simulink model "CART3_FAC"  (R2020a)
settings: Solver=ode4  StartTime=0.0  StopTime=TMax  FixedStep=DT  MaxStep=DT  RelTol=1e-3
InitFcn:
  | run('C:\Users\banderso2\Documents\MIRACL\CART3_FAC_paper\CART dependencies\CARTinitFcn.m')
model workspace (MAT data in the model file):
  Vnom = 480
  fnom = 60
undefined symbols (not defined in the file or in its folder): cHinfDiscreteSISO, ctrl, DiscIntNeverNeededParam, DT, GenEff, OutList, strmatch, timer
libraries: cstblocks x7, discretizing x7, powerlib_meascontrol x1
settings Model: Creator=bjonkman  LastModifiedBy=banderso2
settings DataIOCC: LimitDataPoints=on  SaveFormat=Array  SignalLoggingSaveFormat=ModelDataLogs  SaveOutput=off  SaveTime=off  ReturnWorkspaceOutputs=off  SignalLoggingName=sigsOut
settings OptimizationCC: ExpressionDepthLimit=2147483647  LifeSpan=inf
settings DebuggingCC: SaveWithParameterizedLinksMsg=none  MergeDetectMultiDrivingBlocksExec=none  SignalResolutionControl=TryResolveAllWithWarning  MultiTaskDSMMsg=warning  MultiTaskCondExecSysMsg=none  FcnCallInpInsideContextMsg=warning  StateNameClashWarn=warning  SFUnexpectedBacktrackingDiag=warning  SFNoUnconditionalDefaultTransitionDiag=warning  SFExecutionAtInitializationDiag=none  ArithmeticOperatorsInVariantConditions=warning
settings HardwareCC: ProdBitPerPointer=32  ProdBitPerSizeT=32  ProdBitPerPtrDiffT=32  ProdLargestAtomicFloat=None  ProdIntDivRoundTo=Undefined  ProdEndianess=Unspecified  ProdWordSize=32  ProdHWDeviceType=32-bit Generic  TargetUnknown=on
settings ModelReferenceCC: PropagateSignalLabelsOutOfModel=off
settings SFSimCC: SimUseLocalCustomCode=off  CustomCodeUndefinedFunction=UseInterfaceOnly
settings RTWCC: RTWUseLocalCustomCode=off
settings CodeAppCC: StateflowObjectComments=on
settings GRTTargetCC: TargetLangStandard=C89/C90 (ANSI)  CombineOutputUpdateFcns=off  GRTInterface=on
settings ConfigComp: CovMetricSettings=dw  CovHtmlReporting=on  CovSaveCumulativeToWorkspaceVar=on  CovSaveSingleToWorkspaceVar=on  CovExternalEMLEnable=off

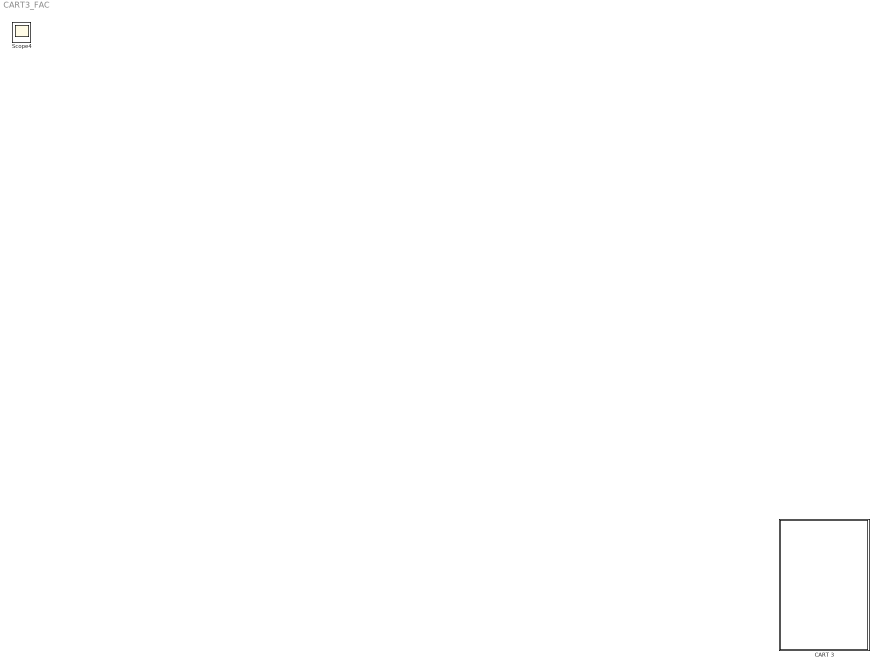
== system CART3_FAC ==
  CART 3 : Subsystem
      mask Display: image('C:\Users\banderso2\Pictures\Saved Pictures\CART3.png'); % Use "Edit Image" on toolstrip to change.
  Scope4 : Scope

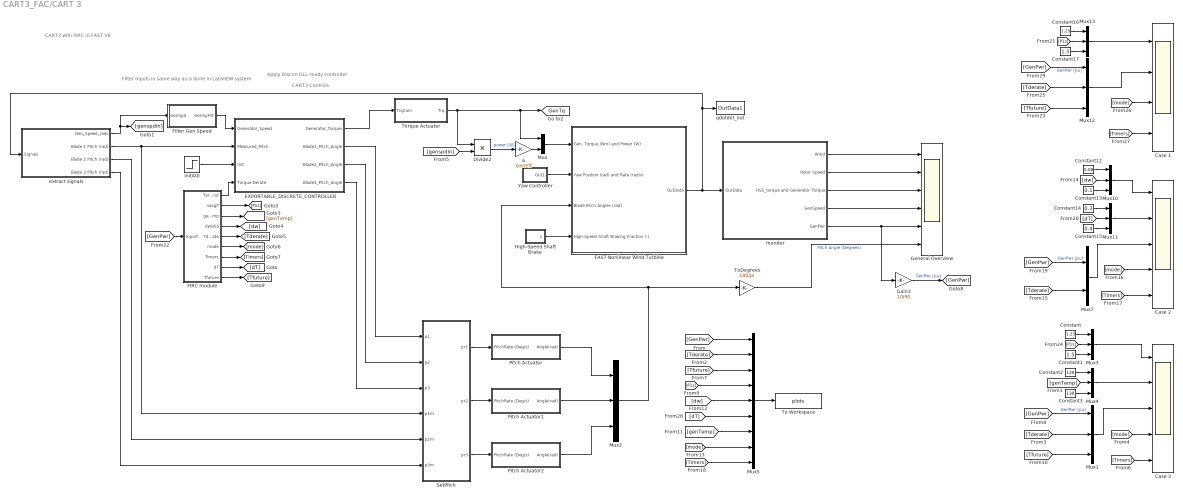
== system CART3_FAC/CART 3 ==
  note: Filter inputs in same way as is done in LabVIEW system
  note: CART3 with FIRC in FAST V8
  note: CART3 Controls
  note: Apply Discon DLL ready controller
  "Case 1 " : Scope  NumInputPorts=4
  Case 2 : Scope  NumInputPorts=5
  Case 3 : Scope  NumInputPorts=5
  Constant : Constant  Value=1.25
  Constant1 : Constant  Value=1.5
  Constant12 : Constant  Value=0.08
  Constant13 : Constant  Value=0.1
  Constant14 : Constant  Value=0.3
  Constant15 : Constant  Value=0.4
  Constant16 : Constant  Value=1.25
  Constant17 : Constant  Value=1.5
  Constant2 : Constant  Value=120
  Constant3 : Constant  Value=130
  Divide2 : Product  Inputs=**
  EXPORTABLE_DISCRETE_CONTROLLER : Subsystem  TreatAsAtomicUnit=on
  FAST Nonlinear Wind Turbine : Subsystem  mask(FAST Nonlinear Wind Turbine){}
      mask help: This block contains the FAST S-Function.
      mask init:
      | clear FAST_SFunc
  "FIRC module " : Subsystem  SystemSampleTime=DT
  Filter Gen Speed : Subsystem  TreatAsAtomicUnit=on
  Gain3 : Gain  Gain=1/590
  General Overview : Scope  NumInputPorts=6
  High-Speed Shaft Brake : Subsystem
  InitAt0 : Step  Time=1/400  SampleTime=DT
  Mux : Mux  Inputs=2
  Mux{1..4,10..13} (8 alike) : Mux  Inputs=3
  Mux5 : Mux  Inputs=9
  Mux7 : Mux  Inputs=2
  Pitch Actuator : Subsystem  TreatAsAtomicUnit=on  SystemSampleTime=DT
  Pitch Actuator1 : Subsystem  TreatAsAtomicUnit=on
  Pitch Actuator2 : Subsystem  TreatAsAtomicUnit=on
  SetPitch : MATLAB Function  TreatAsAtomicUnit=on
  To Workspace : ToWorkspace  VariableName=plots  SaveFormat=Timeseries  SampleTime=-1
  ToDegrees : Gain  Gain=180/pi
  Torque Actuator : Subsystem  TreatAsAtomicUnit=on
  Yaw Controller : Subsystem
  a : Gain  Gain=GenEff
  extract signals : Subsystem
  monitor : Subsystem
  qdotdot_out : ToWorkspace  VariableName=OutData1  SampleTime=-1
  tag scope: GenTq=global
  wires:
  Mux1/1 -> Case 3/3
  "FIRC module "/3(genTemp) -> [genTemp]
  "FIRC module "/5(Tderate) -> [Tderate]
  Divide2/1 -> a/1  "power [W]"
  Yaw Controller/1(Out1) -> FAST Nonlinear Wind Turbine/2(Yaw Position (rad) and Rate (rad/s))
  EXPORTABLE_DISCRETE_CONTROLLER/3(Blade2_Pitch_Angle) -> SetPitch/2(p2)
  Pitch Actuator/1(Angle(rad)) -> Mux2/1
  extract signals/1(Gen_Speed_rads) -> [genspdin], Filter Gen Speed/1(GenSpd)
  ToDegrees/1 -> General Overview/6  "Pitch Angle (Degrees)"
  FAST Nonlinear Wind Turbine/1(OutData) -> monitor/1(OutData), extract signals/1(Signals), qdotdot_out/1
  monitor/4(GenSpeed) -> General Overview/4
  Mux2/1 -> FAST Nonlinear Wind Turbine/3(Blade Pitch Angles (rad)), ToDegrees/1
  SetPitch/2(pr2) -> Pitch Actuator1/1(PitchRate (Deg/s))
  EXPORTABLE_DISCRETE_CONTROLLER/1(Generator_Torque) -> Torque Actuator/1(TrqCom)
  "FIRC module "/4(dwHSS) -> [dw]
  [genspdin] -> Divide2/2
  Pitch Actuator2/1(Angle(rad)) -> Mux2/3
  High-Speed Shaft Brake/1(Out1) -> FAST Nonlinear Wind Turbine/4(High-Speed Shaft Braking Fraction (-))
  SetPitch/3(pr3) -> Pitch Actuator2/1(PitchRate (Deg/s))
  Pitch Actuator1/1(Angle(rad)) -> Mux2/2
  [Timers] -> Case 3/5
  extract signals/2(Blade 1 Pitch (rad)) -> EXPORTABLE_DISCRETE_CONTROLLER/2(Measured_Pitch), SetPitch/4(p1m)
  [mode] -> Case 3/4
  "FIRC module "/6(mode) -> [mode]
  "FIRC module "/2(savgP) -> [P1s]
  EXPORTABLE_DISCRETE_CONTROLLER/2(Blade1_Pitch_Angle) -> SetPitch/1(p1)
  Filter Gen Speed/1(GenSpFilt) -> EXPORTABLE_DISCRETE_CONTROLLER/1(Generator_Speed)
  EXPORTABLE_DISCRETE_CONTROLLER/4(Blade3_Pitch_Angle) -> SetPitch/3(p3)
  Torque Actuator/1(Trq) -> Divide2/1, Mux/1, [GenTq]
  "FIRC module "/1(Torque Command) -> EXPORTABLE_DISCRETE_CONTROLLER/4(Torque Derate)
  "FIRC module "/7(Timers) -> [Timers]
  SetPitch/1(pr1) -> Pitch Actuator/1(PitchRate (Deg/s))
  monitor/3(HSS_torque and Generator Torque) -> General Overview/3
  a/1 -> Mux/2
  monitor/5(GenPwr) -> Gain3/1, General Overview/5
  Mux/1 -> FAST Nonlinear Wind Turbine/1(Gen. Torque (Nm) and Power (W))
  monitor/1(Wind) -> General Overview/1
  InitAt0/1 -> EXPORTABLE_DISCRETE_CONTROLLER/3(Init)
  monitor/2(Rotor Speed) -> General Overview/2
  extract signals/4(Blade 3 Pitch (rad)) -> SetPitch/6(p3m)
  extract signals/3(Blade 2 Pitch (rad)) -> SetPitch/5(p2m)
  "FIRC module "/8(dT) -> [dT]
  Constant/1 -> Mux3/1
  Constant1/1 -> Mux3/3
  Constant2/1 -> Mux4/1
  [genTemp] -> Mux4/2
  Constant3/1 -> Mux4/3
  "FIRC module "/9(Tfuture) -> [Tfuture]
  Mux3/1 -> Case 3/1
  [GenPwr] -> Mux1/1  "GenPwr [pu]"
  [Tderate] -> Mux1/2
  [Tfuture] -> Mux1/3
  Mux11/1 -> Case 2/2
  [Tderate] -> Mux7/2
  [GenPwr] -> Mux7/1  "GenPwr [pu]"
  Constant13/1 -> Mux10/3
  Constant12/1 -> Mux10/1
  Mux7/1 -> Case 2/3
  Constant14/1 -> Mux11/1
  [dw] -> Mux10/2
  [dT] -> Mux11/2
  [Timers] -> Case 2/5
  Constant15/1 -> Mux11/3
  [mode] -> Case 2/4
  Mux10/1 -> Case 2/1
  [Timers] -> "Case 1 "/4
  [Tderate] -> Mux12/2
  [Tfuture] -> Mux12/3
  Mux13/1 -> "Case 1 "/1
  [GenPwr] -> Mux12/1  "GenPwr [pu]"
  Mux12/1 -> "Case 1 "/2
  [mode] -> "Case 1 "/3
  Constant16/1 -> Mux13/1
  [P1s] -> Mux13/2
  Constant17/1 -> Mux13/3
  Mux4/1 -> Case 3/2
  [GenPwr] -> "FIRC module "/1(Inport)
  [P1s] -> Mux3/2
  Gain3/1 -> [GenPwr]  "GenPwr [pu]"
  [GenPwr] -> Mux5/1
  [Tderate] -> Mux5/2
  [Tfuture] -> Mux5/3
  [P1s] -> Mux5/4
  [dw] -> Mux5/5
  [dT] -> Mux5/6
  [genTemp] -> Mux5/7
  [mode] -> Mux5/8
  [Timers] -> Mux5/9
  Mux5/1 -> To Workspace/1

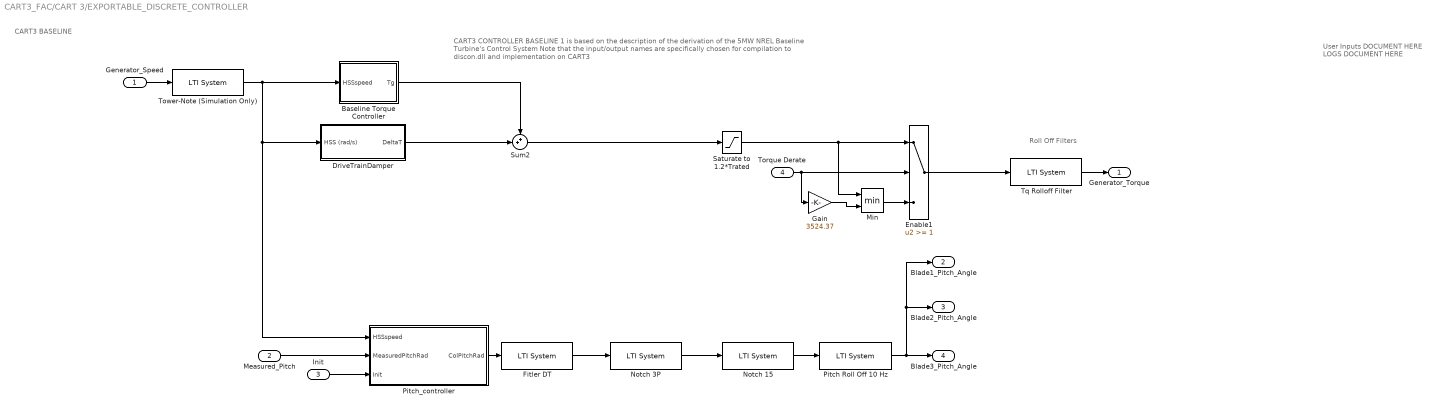
== system CART3_FAC/CART 3/EXPORTABLE_DISCRETE_CONTROLLER ==
  note: CART3 CONTROLLER BASELINE 1 is based on the description of the derivation of the 5MW NREL Baseline Turbine's Control System
      | Note that the input/output names are specifically chosen for compilation to discon.dll and implementation on CART3
  note: Roll Off Filters
  note: User Inputs
      | DOCUMENT HERE
      |
      | LOGS
      | DOCUMENT HERE
  note: CART3 BASELINE
  Generator_Speed : Inport
  Measured_Pitch : Inport  Port=2  PortDimensions=1
  Init : Inport  Port=3  PortDimensions=1
  Torque Derate : Inport  Port=4  PortDimensions=1
  Baseline Torque Controller : Subsystem
  DriveTrainDamper : Subsystem  TreatAsAtomicUnit=on
  Enable1 : Switch  Threshold=1
  Fitler DT : cstblocks/LTI System  sys=FilterDTAdj  IC=[]
  Gain : Gain  Gain=3524.37
  Min : MinMax  Inputs=2
  Notch 15 : cstblocks/LTI System  sys=Notch15  IC=[]
  Notch 3P : cstblocks/LTI System  sys=Notch3PAdj  IC=[]
  Pitch Roll Off 10 Hz : cstblocks/LTI System  sys=PitchRolloff10Hz  IC=[]
  Pitch_controller : Subsystem
  Saturate to 1.2*Trated : Saturate  UpperLimit=1.2*3.5296e+003  LowerLimit=100
  Sum2 : Sum  Inputs=++|
  Tower-Note (Simulation Only) : cstblocks/LTI System  sys=Gen_p9Hz_Notch  IC=[]
  Tq Rolloff Filter : cstblocks/LTI System  sys=TqFilt  IC=[]
  Generator_Torque : Outport
  Blade1_Pitch_Angle : Outport  Port=2  PortDimensions=1
  Blade2_Pitch_Angle : Outport  Port=3  PortDimensions=1
  Blade3_Pitch_Angle : Outport  Port=4  PortDimensions=1
  wires:
  Init/1 -> Pitch_controller/3(Init)
  Generator_Speed/1 -> Tower-Note (Simulation Only)/1
  Fitler DT/1 -> Notch 3P/1
  Notch 3P/1 -> Notch 15/1
  Notch 15/1 -> Pitch Roll Off 10 Hz/1
  Pitch Roll Off 10 Hz/1 -> Blade1_Pitch_Angle/1, Blade2_Pitch_Angle/1, Blade3_Pitch_Angle/1
  Tq Rolloff Filter/1 -> Generator_Torque/1
  Measured_Pitch/1 -> Pitch_controller/2(MeasuredPitchRad)
  Pitch_controller/1(ColPitchRad) -> Fitler DT/1
  Tower-Note (Simulation Only)/1 -> Baseline Torque Controller/1(HSSspeed), Pitch_controller/1(HSSspeed), DriveTrainDamper/1(HSS (rad/s))
  DriveTrainDamper/1(DeltaT) -> Sum2/2
  Baseline Torque Controller/1(Tg) -> Sum2/1
  Sum2/1 -> Saturate to 1.2*Trated/1
  Torque Derate/1 -> Enable1/2, Gain/1
  Saturate to 1.2*Trated/1 -> Min/1, Enable1/1
  Min/1 -> Enable1/3
  Gain/1 -> Min/2
  Enable1/1 -> Tq Rolloff Filter/1

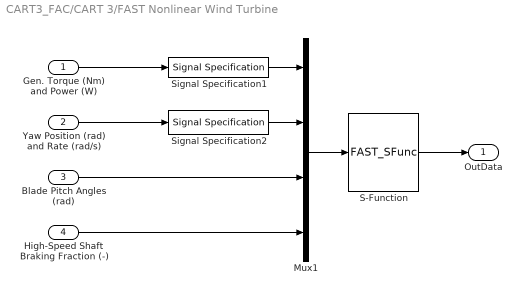
== system CART3_FAC/CART 3/FAST Nonlinear Wind Turbine ==
  Gen. Torque (Nm) and Power (W) : Inport
  Yaw Position (rad) and Rate (rad/s) : Inport  Port=2
  Blade Pitch Angles (rad) : Inport  Port=3
  High-Speed Shaft Braking Fraction (-) : Inport  Port=4
  Mux1 : Mux
  S-Function : S-Function  FunctionName=FAST_SFunc  Parameters=FAST_InputFileName, TMax, 0  SFunctionDeploymentMode=off  EnableBusSupport=off
  Signal Specification1 : SignalSpecification  OutDataTypeStr=double  Dimensions=2
  Signal Specification2 : SignalSpecification  OutDataTypeStr=double  Dimensions=2
  OutData : Outport
  wires:
  Gen. Torque (Nm) and Power (W)/1 -> Signal Specification1/1
  S-Function/1 -> OutData/1
  Mux1/1 -> S-Function/1
  Blade Pitch Angles (rad)/1 -> Mux1/3
  Yaw Position (rad) and Rate (rad/s)/1 -> Signal Specification2/1
  Signal Specification1/1 -> Mux1/1
  Signal Specification2/1 -> Mux1/2
  High-Speed Shaft Braking Fraction (-)/1 -> Mux1/4

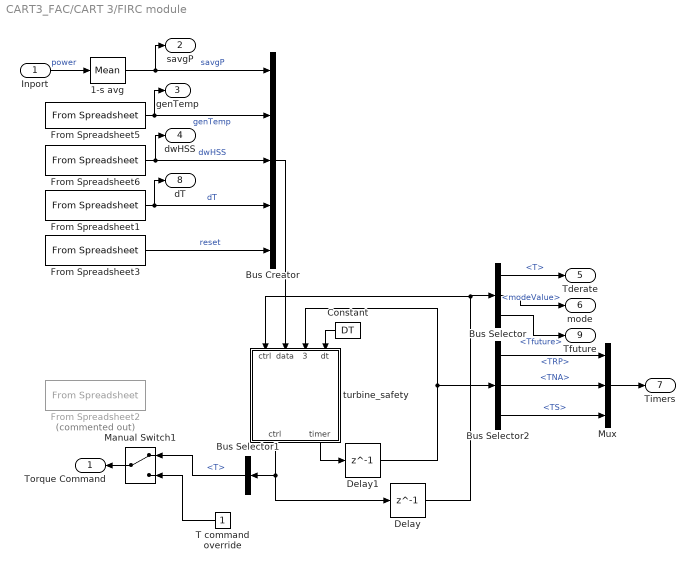
== system CART3_FAC/CART 3/FIRC module  ==
  Inport : Inport
  1-s avg : powerlib_meascontrol/Measurements/Mean  Freq=1  Vinit=0  Ts=0
  Bus Creator : BusCreator  Inputs=5
  Bus Selector : BusSelector  OutputSignals=T,modeValue,Tfuture
  Bus Selector1 : BusSelector  OutputSignals=T
  Bus Selector2 : BusSelector  OutputSignals=TRP,TNA,TS
  Constant : Constant  Value=DT
  Delay : Delay  DelayLength=1  InitialCondition=ctrl
  Delay1 : Delay  DelayLength=1  InitialCondition=timer
  From Spreadsheet1 : FromSpreadsheet  FileName=fault_timeseries.xlsx  SheetName=dT  SampleTime=DT
  From Spreadsheet2 : FromSpreadsheet  Commented=on  FileName=fault_timeseries.xlsx  SheetName=ax  SampleTime=DT
  From Spreadsheet3 : FromSpreadsheet  FileName=fault_timeseries.xlsx  SheetName=reset  SampleTime=DT
  From Spreadsheet5 : FromSpreadsheet  FileName=fault_timeseries.xlsx  SheetName=genTemp  SampleTime=DT
  From Spreadsheet6 : FromSpreadsheet  FileName=fault_timeseries.xlsx  SheetName=dwHSS  SampleTime=DT
  Manual Switch1 : ManualSwitch
  Mux : Mux  Inputs=3
  T command override : Constant
  "turbine_safety " : MATLAB Function  TreatAsAtomicUnit=on
  Torque Command : Outport
  savgP : Outport  Port=2
  genTemp : Outport  Port=3
  dwHSS : Outport  Port=4
  Tderate : Outport  Port=5
  mode : Outport  Port=6
  Timers : Outport  Port=7
  dT : Outport  Port=8
  Tfuture : Outport  Port=9
  wires:
  From Spreadsheet5/1 -> genTemp/1, Bus Creator/2  "genTemp"
  Manual Switch1/1 -> Torque Command/1
  "turbine_safety "/1(ctrl) -> Delay/1, Bus Selector1/1
  Delay1/1 -> "turbine_safety "/3("timer "), Bus Selector2/1
  Delay/1 -> "turbine_safety "/1("ctrl "), Bus Selector/1
  "turbine_safety "/2(timer) -> Delay1/1
  From Spreadsheet6/1 -> dwHSS/1, Bus Creator/3  "dwHSS"
  Bus Creator/1 -> "turbine_safety "/2(data)
  T command override/1 -> Manual Switch1/2
  Bus Selector1/1 -> Manual Switch1/1  "<T>"
  Inport/1 -> 1-s avg/1  "power"
  Bus Selector/2 -> mode/1  "<modeValue>"
  Bus Selector2/1 -> Mux/1  "<TRP>"
  Bus Selector/1 -> Tderate/1  "<T>"
  Mux/1 -> Timers/1
  Constant/1 -> "turbine_safety "/4(dt)
  Bus Selector2/2 -> Mux/2  "<TNA>"
  From Spreadsheet1/1 -> Bus Creator/4, dT/1  "dT"
  Bus Selector2/3 -> Mux/3  "<TS>"
  Bus Selector/3 -> Tfuture/1  "<Tfuture>"
  1-s avg/1 -> savgP/1, Bus Creator/1  "savgP"
  From Spreadsheet3/1 -> Bus Creator/5  "reset"

== system CART3_FAC/CART 3/Filter Gen Speed ==
  GenSpd : Inport
  HSS Filter : MATLAB Function  TreatAsAtomicUnit=on
  Unit Delay : UnitDelay  SampleTime=-1  HasFrameUpgradeWarning=on
  GenSpFilt : Outport
  wires:
  HSS Filter/1(y) -> Unit Delay/1, GenSpFilt/1
  Unit Delay/1 -> HSS Filter/2(z)
  GenSpd/1 -> HSS Filter/1(u)

== system CART3_FAC/CART 3/High-Speed Shaft Brake ==
  High-Speed Shaft Braking Fraction : Constant  Value=0
  Out1 : Outport
  wires:
  High-Speed Shaft Braking Fraction/1 -> Out1/1

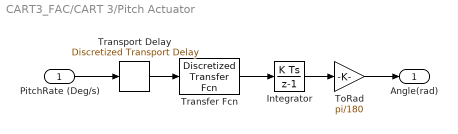
== system CART3_FAC/CART 3/Pitch Actuator ==
  PitchRate (Deg/s) : Inport
  Integrator : DiscreteIntegrator  SampleTime=0.0025  ICPrevOutput=DiscIntNeverNeededParam  ICPrevScaledInput=DiscIntNeverNeededParam  mask(DiscretizedDiscreteIntegrator){}
      mask init:
      | %zoh
  ToRad : Gain  Gain=pi/180
  Transfer Fcn : discretizing/Discretized Transfer Fcn  Numerator=[60]  Denominator=[1 60]  AbsTol=auto  SampleTime=0.0025  method=zoh  Wc=1
      settings: SourceProductBaseCode=SL
  Transport Delay : discretizing/Discretized Transport Delay  delay=0.015  ic=0  SampleTime=0.0025  rounding=Floor
      settings: SourceProductBaseCode=SL
  Angle(rad) : Outport
  wires:
  PitchRate (Deg/s)/1 -> Transport Delay/1
  Transport Delay/1 -> Transfer Fcn/1
  Transfer Fcn/1 -> Integrator/1
  Integrator/1 -> ToRad/1
  ToRad/1 -> Angle(rad)/1

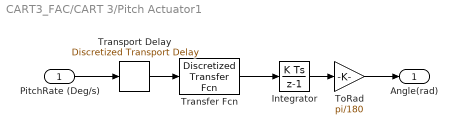
== system CART3_FAC/CART 3/Pitch Actuator1 ==
  PitchRate (Deg/s) : Inport
  Integrator : DiscreteIntegrator  SampleTime=0.0025  ICPrevOutput=DiscIntNeverNeededParam  ICPrevScaledInput=DiscIntNeverNeededParam  mask(DiscretizedDiscreteIntegrator){}
      mask init:
      | %zoh
  ToRad : Gain  Gain=pi/180
  Transfer Fcn : discretizing/Discretized Transfer Fcn  Numerator=[60]  Denominator=[1 60]  AbsTol=auto  SampleTime=0.0025  method=zoh  Wc=1
      settings: SourceProductBaseCode=SL
  Transport Delay : discretizing/Discretized Transport Delay  delay=0.015  ic=0  SampleTime=0.0025  rounding=Floor
      settings: SourceProductBaseCode=SL
  Angle(rad) : Outport
  wires:
  ToRad/1 -> Angle(rad)/1
  Integrator/1 -> ToRad/1
  Transfer Fcn/1 -> Integrator/1
  Transport Delay/1 -> Transfer Fcn/1
  PitchRate (Deg/s)/1 -> Transport Delay/1

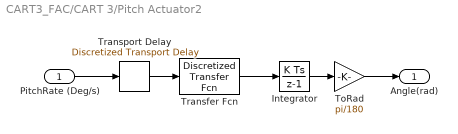
== system CART3_FAC/CART 3/Pitch Actuator2 ==
  PitchRate (Deg/s) : Inport
  Integrator : DiscreteIntegrator  SampleTime=0.0025  ICPrevOutput=DiscIntNeverNeededParam  ICPrevScaledInput=DiscIntNeverNeededParam  mask(DiscretizedDiscreteIntegrator){}
      mask init:
      | %zoh
  ToRad : Gain  Gain=pi/180
  Transfer Fcn : discretizing/Discretized Transfer Fcn  Numerator=[60]  Denominator=[1 60]  AbsTol=auto  SampleTime=0.0025  method=zoh  Wc=1
      settings: SourceProductBaseCode=SL
  Transport Delay : discretizing/Discretized Transport Delay  delay=0.015  ic=0  SampleTime=0.0025  rounding=Floor
      settings: SourceProductBaseCode=SL
  Angle(rad) : Outport
  wires:
  ToRad/1 -> Angle(rad)/1
  Integrator/1 -> ToRad/1
  Transfer Fcn/1 -> Integrator/1
  Transport Delay/1 -> Transfer Fcn/1
  PitchRate (Deg/s)/1 -> Transport Delay/1

== system CART3_FAC/CART 3/Torque Actuator ==
  TrqCom : Inport
  Transport Delay : discretizing/Discretized Transport Delay  delay=0.05  ic=0  SampleTime=0.0025  rounding=Floor
      settings: SourceProductBaseCode=SL
  Trq : Outport
  wires:
  TrqCom/1 -> Transport Delay/1
  Transport Delay/1 -> Trq/1

== system CART3_FAC/CART 3/Yaw Controller ==
  Mux : Mux  Inputs=2
  Yaw Position : Constant  Value=0
  Yaw rate : Constant  Value=0
  Out1 : Outport
  wires:
  Mux/1 -> Out1/1
  Yaw Position/1 -> Mux/1
  Yaw rate/1 -> Mux/2

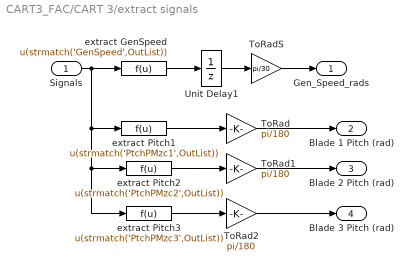
== system CART3_FAC/CART 3/extract signals ==
  Signals : Inport
  ToRad : Gain  Gain=pi/180
  ToRad1 : Gain  Gain=pi/180
  ToRad2 : Gain  Gain=pi/180
  ToRadS : Gain  Gain=pi/30
  Unit Delay1 : UnitDelay  InitialCondition=12.1*97  SampleTime=DT  HasFrameUpgradeWarning=on
  extract GenSpeed : Fcn  Expr=u(strmatch('GenSpeed',OutList))
  extract Pitch1 : Fcn  Expr=u(strmatch('PtchPMzc1',OutList))
  extract Pitch2 : Fcn  Expr=u(strmatch('PtchPMzc2',OutList))
  extract Pitch3 : Fcn  Expr=u(strmatch('PtchPMzc3',OutList))
  Gen_Speed_rads : Outport
  Blade 1 Pitch (rad) : Outport  Port=2
  Blade 2 Pitch (rad) : Outport  Port=3
  Blade 3 Pitch (rad) : Outport  Port=4
  wires:
  extract GenSpeed/1 -> Unit Delay1/1
  Signals/1 -> extract GenSpeed/1, extract Pitch1/1, extract Pitch2/1, extract Pitch3/1
  Unit Delay1/1 -> ToRadS/1
  ToRadS/1 -> Gen_Speed_rads/1
  extract Pitch1/1 -> ToRad/1
  extract Pitch2/1 -> ToRad1/1
  extract Pitch3/1 -> ToRad2/1
  ToRad2/1 -> Blade 3 Pitch (rad)/1
  ToRad1/1 -> Blade 2 Pitch (rad)/1
  ToRad/1 -> Blade 1 Pitch (rad)/1

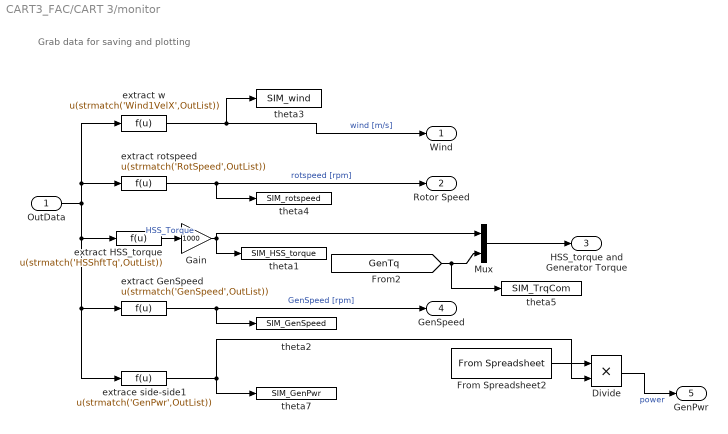
== system CART3_FAC/CART 3/monitor ==
  note: Grab data for saving and plotting
  OutData : Inport
  Divide : Product  Inputs=**
  From Spreadsheet2 : FromSpreadsheet  FileName=fault_timeseries.xlsx  SheetName=power_multiplier  SampleTime=DT
  Gain : Gain  Gain=1000
  Mux : Mux  Inputs=2
  extrace side-side1 : Fcn  Expr=u(strmatch('GenPwr',OutList))
  extract GenSpeed : Fcn  Expr=u(strmatch('GenSpeed',OutList))
  extract HSS_torque : Fcn  Expr=u(strmatch('HSShftTq',OutList))
  extract rotspeed : Fcn  Expr=u(strmatch('RotSpeed',OutList))
  extract w : Fcn  Expr=u(strmatch('Wind1VelX',OutList))
  theta1 : ToWorkspace  VariableName=SIM_HSS_torque  SampleTime=-1
      settings: MaxDataPoints=Inf  Decimation=10
  theta2 : ToWorkspace  VariableName=SIM_GenSpeed  SampleTime=-1
      settings: MaxDataPoints=Inf  Decimation=10
  theta3 : ToWorkspace  VariableName=SIM_wind  SampleTime=-1
      settings: MaxDataPoints=Inf  Decimation=10
  theta4 : ToWorkspace  VariableName=SIM_rotspeed  SampleTime=-1
      settings: MaxDataPoints=Inf  Decimation=10
  theta5 : ToWorkspace  VariableName=SIM_TrqCom  SampleTime=-1
      settings: MaxDataPoints=Inf  Decimation=10
  theta7 : ToWorkspace  VariableName=SIM_GenPwr  SampleTime=-1
      settings: MaxDataPoints=Inf  Decimation=10
  Wind : Outport
  Rotor Speed : Outport  Port=2
  HSS_torque and Generator Torque : Outport  Port=3
  GenSpeed : Outport  Port=4
  GenPwr : Outport  Port=5
  wires:
  extract w/1 -> theta3/1, Wind/1  "wind [m/s]"
  extract rotspeed/1 -> theta4/1, Rotor Speed/1  "rotspeed [rpm]"
  extract HSS_torque/1 -> Gain/1  "HSS_Torque"
  extract GenSpeed/1 -> theta2/1, GenSpeed/1  "GenSpeed [rpm]"
  [GenTq] -> Mux/2, theta5/1
  Mux/1 -> HSS_torque and Generator Torque/1
  Gain/1 -> theta1/1, Mux/1
  extrace side-side1/1 -> Divide/2, theta7/1
  OutData/1 -> extract rotspeed/1, extract w/1, extract HSS_torque/1, extract GenSpeed/1, extrace side-side1/1
  From Spreadsheet2/1 -> Divide/1
  Divide/1 -> GenPwr/1  "power"

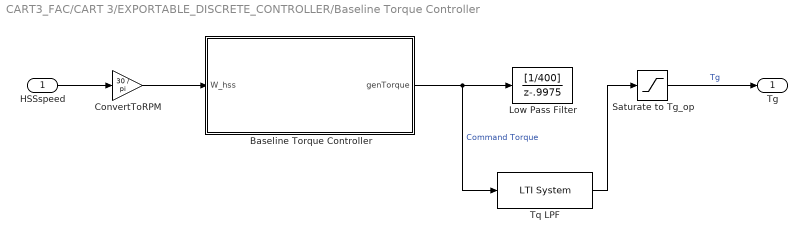
== system CART3_FAC/CART 3/EXPORTABLE_DISCRETE_CONTROLLER/Baseline Torque Controller ==
  HSSspeed : Inport
  Baseline Torque Controller : MATLAB Function  TreatAsAtomicUnit=on
  ConvertToRPM : Gain  Gain=30 / pi
  Low Pass Filter : DiscreteTransferFcn  Numerator=[1/400]  Denominator=[1 -.9975]  SampleTime=1/400
  Saturate to Tg_op : Saturate  UpperLimit=3524.36  LowerLimit=0
  Tq LPF : cstblocks/LTI System  sys=TqLPF  IC=[]
  Tg : Outport
  wires:
  Baseline Torque Controller/1(genTorque) -> Low Pass Filter/1, Tq LPF/1  "Command Torque"
  HSSspeed/1 -> ConvertToRPM/1
  ConvertToRPM/1 -> Baseline Torque Controller/1(W_hss)
  Saturate to Tg_op/1 -> Tg/1  "Tg"
  Tq LPF/1 -> Saturate to Tg_op/1

== system CART3_FAC/CART 3/EXPORTABLE_DISCRETE_CONTROLLER/DriveTrainDamper ==
  HSS (rad/s) : Inport
  ConvertToRadians : Gain  Gain=pi / 30
  HinfDriveTrainDamper : DiscreteStateSpace  A=cHinfDiscreteSISO.A  B=cHinfDiscreteSISO.B  C=cHinfDiscreteSISO.C  D=cHinfDiscreteSISO.D  SampleTime=DT
  MAXRPM : Constant  Value=1600
  Sum : Sum  Inputs=|+-
  DeltaT : Outport
  wires:
  HSS (rad/s)/1 -> Sum/2
  Sum/1 -> HinfDriveTrainDamper/1
  HinfDriveTrainDamper/1 -> DeltaT/1
  MAXRPM/1 -> ConvertToRadians/1
  ConvertToRadians/1 -> Sum/1

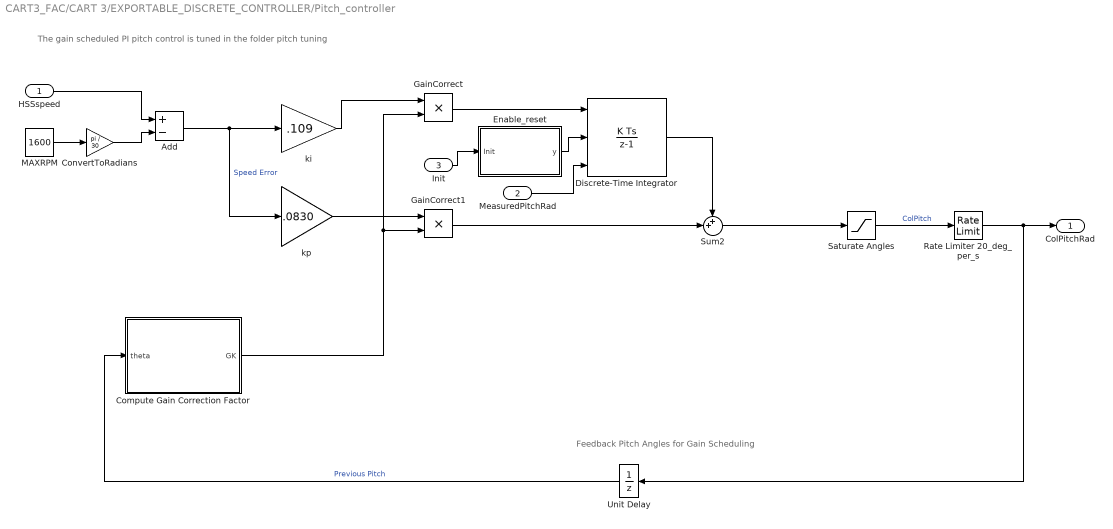
== system CART3_FAC/CART 3/EXPORTABLE_DISCRETE_CONTROLLER/Pitch_controller ==
  note: Feedback Pitch Angles for Gain Scheduling
  note: The gain scheduled PI pitch control is tuned in the folder pitch tuning
  HSSspeed : Inport
  MeasuredPitchRad : Inport  Port=2
  Init : Inport  Port=3
  Add : Sum  Inputs=+-
  Compute Gain Correction Factor : MATLAB Function  TreatAsAtomicUnit=on
  ConvertToRadians : Gain  Gain=pi / 30
  Discrete-Time Integrator : DiscreteIntegrator  gainval=1  ExternalReset=level  InitialConditionSource=external  InitialCondition=3.7*pi/180  SampleTime=1/400  LimitOutput=on  UpperSaturationLimit=pi/2  LowerSaturationLimit=3.7*pi/180  ICPrevOutput=DiscIntNeverNeededParam  ICPrevScaledInput=DiscIntNeverNeededParam
  Enable_reset : MATLAB Function  TreatAsAtomicUnit=on
  GainCorrect : Product  RndMeth=Zero
  GainCorrect1 : Product  RndMeth=Zero
  MAXRPM : Constant  Value=1600
  Rate Limiter 20_deg_per_s : RateLimiter  RisingSlewLimit=20 * pi / 180  FallingSlewLimit=-20 * pi /180  SampleTimeMode=inherited
  Saturate Angles : Saturate  UpperLimit=pi/2  LowerLimit=3.7 * pi / 180
  Sum2 : Sum  Inputs=++|
  Unit Delay : UnitDelay  SampleTime=0.0025  HasFrameUpgradeWarning=on
  ki : Gain  Gain=.109
  kp : Gain  Gain=.0830
  ColPitchRad : Outport
  wires:
  Add/1 -> kp/1, ki/1  "Speed Error"
  Unit Delay/1 -> Compute Gain Correction Factor/1(theta)  "Previous Pitch"
  kp/1 -> GainCorrect1/1
  Compute Gain Correction Factor/1(GK) -> GainCorrect/2, GainCorrect1/2
  GainCorrect1/1 -> Sum2/2
  HSSspeed/1 -> Add/1
  Discrete-Time Integrator/1 -> Sum2/1
  Saturate Angles/1 -> Rate Limiter 20_deg_per_s/1  "ColPitch"
  Rate Limiter 20_deg_per_s/1 -> ColPitchRad/1, Unit Delay/1
  ki/1 -> GainCorrect/1
  MAXRPM/1 -> ConvertToRadians/1
  ConvertToRadians/1 -> Add/2
  MeasuredPitchRad/1 -> Discrete-Time Integrator/3
  Enable_reset/1(y) -> Discrete-Time Integrator/2
  Init/1 -> Enable_reset/1(Init)
  Sum2/1 -> Saturate Angles/1
  GainCorrect/1 -> Discrete-Time Integrator/1

== matlab function CART3_FAC/CART 3/EXPORTABLE_DISCRETE_CONTROLLER/Baseline Torque Controller/Baseline Torque Controller ==
  settings: fimath=|
      | fimath(...
      | 'RoundMode', 'floor',...
      | 'OverflowMode', 'wrap',...
      | 'ProductMode', 'KeepLSB', 'ProductWordLength', 32,...
      | 'SumMode', 'KeepLSB', 'SumWordLength', 32,...
      | 'CastBeforeSum', false)
  data: W_hss input; genTorque output
function genTorque = regionSelectTq(W_hss)
% This function adapted by Paul Fleming from one written by JW van Wingerden
%Currently does not contain any checks on pitch angle for fear
%future advanced codes will trip this accidentally
%
%Also does not contain region 1.5 as documented in Jonkman
%Also does not contain "optimal tracking rotor code"
%See unused Torque Controller Block for example of pitch influence

%Define constants
DENSITY = 1.0; %Measured 10/21/10
RADIUS = 20;
CPZERO = .4658;
TSRZERO = 7.1; %Higher TSR to get rid of awkward saturation region 2.5
MAXTORQUE = 3524.37;
RATIO = 43.164;
MAXRPM = 1600; %lowered RPM for stability

%Calculate k
K = ((DENSITY*pi* RADIUS^5*CPZERO)/ (2.0*TSRZERO^3));


%Region 2
genTorque = K / (RATIO^3) * (W_hss * pi / 30) ^2;

%Region 2.5 Code
if((MAXTORQUE/(MAXRPM*0.05))*(W_hss-MAXRPM*0.92) > genTorque)
    genTorque = (MAXTORQUE/(MAXRPM*0.05))*(W_hss-MAXRPM*0.92);
end

%Region 3 code
if ( genTorque > MAXTORQUE || W_hss > 0.99 * MAXRPM)
    genTorque = MAXTORQUE;
end



%Region 1
if (W_hss < 10 * RATIO)
    genTorque = 0;
end

%m1_5= K*520^2/120;          %Region 2.5 slope (Nm/rpm)
%c1_5 = -K*520^2/120*400;     %Region 2.5 offset (Nm)
%elseif (W_hss > 400)                    %Region 1.5
%    genTorque = m1_5 * W_hss + c1_5;

== matlab function CART3_FAC/CART 3/EXPORTABLE_DISCRETE_CONTROLLER/Pitch_controller/Compute Gain Correction Factor ==
  settings: fimath=|
      | fimath(...
      | 'RoundMode', 'floor',...
      | 'OverflowMode', 'wrap',...
      | 'ProductMode', 'KeepLSB', 'ProductWordLength', 32,...
      | 'SumMode', 'KeepLSB', 'SumWordLength', 32,...
      | 'CastBeforeSum', false)
  data: theta input; GK output
function GK = computeGain(theta)
% This function computed the gain correction as described in
% J. Jonkman, S. Butterfield, W. Musial, and G. Scott, Definition of a 5-MW Reference Wind Turbine for Offshore System Development Definition of a 5-MW Reference Wind Turbine for Offshore System Development, 2009.

%Define constants
thetaK = 3.0895 * pi / 180;

GK = 1 / ( 1 + (theta / thetaK));

== matlab function CART3_FAC/CART 3/EXPORTABLE_DISCRETE_CONTROLLER/Pitch_controller/Enable_reset ==
  settings: fimath=|
      | fimath(...
      | 'RoundMode', 'floor',...
      | 'OverflowMode', 'wrap',...
      | 'ProductMode', 'KeepLSB', 'ProductWordLength', 32,...
      | 'SumMode', 'KeepLSB', 'SumWordLength', 32,...
      | 'CastBeforeSum', false)
  data: Init input; y output
function y = reset(Init)


if Init>0.9 && Init<1.1
    y=0;
else
    y=1;
end

== matlab function CART3_FAC/CART 3/FIRC module /turbine_safety  ==
  data: ctrl input Bus: ctrlBus; data input Bus: dataBus; ctrl output; timer input Bus: timerBus; timer output; faulty parameter; dt input
 function [ctrl, timer]   = turbine_safety(ctrl, data, timer, faulty, dt)
    % Fault adaptive controller. Checks various sensor readings, and
    % responds by entering the appropriate control mode, providing the
    % appropriate torque derate, and setting the appropriate timers.
    [timer,ctrl] = checkReset(ctrl, timer, data);      
    % if faulted, don't change anything 
    if ctrl.mode(4)+ctrl.mode(5)+ctrl.mode(6) == 0 %if not faulted
        ctrl.RP_prev = ctrl.mode(2); %0 if ctrl.cmd =0; 1 otherwise
        fields = fieldnames(faulty); %run warning logic for all faultys
        ctrl.mode = [0,0,0,0,0,0];
        for i=1:length(fields)
            ctrl.(fields{i}).state = 0;
            checkHandle = str2func(faulty.(fields{i}).checkFun); %check for warnings/faultys
            ctrl = checkHandle(data, ctrl);
            ctrl = setMode(ctrl, faulty, fields{i}); %set mode
        end
        [ctrl, timer] = setTimers(ctrl, timer, dt); %set timers and torque derate
        ctrl.modeValue = sum(ctrl.mode.*2.^linspace(0,5,6));
    else
        if ctrl.mode(6) == 1
            fprintf('EMERGENCY STOP')
        elseif ctrl.mode(5) == 1
            fprintf('OPEN LOOP NORMAL STOP')
        elseif ctrl.mode(4) == 1
            fprintf('NORMAL STOP')
        end

%     displays for testing
%         disp('ctrl.mode:')
%         disp(ctrl.mode)
%         disp('data:')
%         disp(data)
%         disp('timer:')
%         disp(timer)
%         fprintf('data = %1.0f\n', data);
%         fprintf('ctrl.Ttarget = %1.0f\n', ctrl.Ttarget);

    end

== matlab function CART3_FAC/CART 3/Filter Gen Speed/HSS Filter ==
  data: u input; y output; z input
function y = fcn(u,z)
%#eml

Alpha     = exp( ( -0.0025 ) / .025 );
y = ( 1.0 - Alpha )*u + Alpha*z;

== matlab function CART3_FAC/CART 3/SetPitch ==
  data: p1 input; pr1 output; p2 input; p3 input; pr2 output; pr3 output; p1m input; p2m input; p3m input
function [pr1,pr2,pr3] = setpitch(p1, p2, p3, p1m, p2m, p3m)
%#eml

%Note that the m stands for measured in p1m

MAXPITCH = 90;
MINPITCH = -10;
MAXPITCHRATE = 25;

%Convert to degrees
p1 = p1 * 180 / pi;
p2 = p2 * 180 / pi;
p3 = p3 * 180 / pi;
p1m = p1m * 180 / pi;
p2m = p2m * 180 / pi;
p3m = p3m * 180 / pi;

%Coerce
p1 = max(min(p1,MAXPITCH),MINPITCH);
p2 = max(min(p2,MAXPITCH),MINPITCH);
p3 = max(min(p3,MAXPITCH),MINPITCH);

%Compute error
e1 = p1 - p1m;
e2 = p2 - p2m;
e3 = p3 - p3m;

%Apply k = 5;
pr1 = 5 * e1;
pr2 = 5 * e2;
pr3 = 5 * e3;

%Coerce
pr1 = max(min(pr1,MAXPITCHRATE),-1*MAXPITCHRATE);
pr2 = max(min(pr2,MAXPITCHRATE),-1*MAXPITCHRATE);
pr3 = max(min(pr3,MAXPITCHRATE),-1*MAXPITCHRATE);
